simulink model "test_loopback_buf"  (Simulink 6.2)
settings: Solver=ode45  StartTime=0.0  StopTime=4000  RelTol=1e-3
undefined symbols (not defined in the file): Down, Up
libraries: xbsIndex_r3 x1383, xps_library x52, casper_library x37
(part 2 of 8)

== system test_loopback_buf/Feng_sim_complete1 ==
  Concat : xbsIndex_r3/Concat  num_inputs=2  explicit_period=off  period=1  dbl_ovrd=off
  Concat1 : xbsIndex_r3/Concat  num_inputs=3  explicit_period=off  period=1  dbl_ovrd=off
  Constant : xbsIndex_r3/Constant  const=0  equ=P=C  arith_type=Boolean  n_bits=1  bin_pt=0  opselect=C  inp2=PCIN>>17  opr=+  inp1=P  carry=CIN  iostate=0  explicit_period=on  period=1  dbl_ovrd=off
  Constant1 : xbsIndex_r3/Constant  const=1  equ=P=C  arith_type=Boolean  n_bits=1  bin_pt=0  opselect=C  inp2=PCIN>>17  opr=+  inp1=P  carry=CIN  iostate=0  explicit_period=off  period=1  dbl_ovrd=off
  Constant2 : Constant
  Constant3 : xbsIndex_r3/Constant  const=0  equ=P=C  arith_type=Boolean  n_bits=1  bin_pt=0  opselect=C  inp2=PCIN>>17  opr=+  inp1=P  carry=CIN  iostate=0  explicit_period=off  period=1  dbl_ovrd=off
  Constant4 : xbsIndex_r3/Constant  const=0  equ=P=C  arith_type=Unsigned  n_bits=32  bin_pt=0  opselect=C  inp2=PCIN>>17  opr=+  inp1=P  carry=CIN  iostate=0  explicit_period=on  period=1  dbl_ovrd=off
  Constant5 : xbsIndex_r3/Constant  const=0  equ=P=C  arith_type=Unsigned  n_bits=16-2  bin_pt=0  opselect=C  inp2=PCIN>>17  opr=+  inp1=P  carry=CIN  iostate=0  explicit_period=on  period=1  dbl_ovrd=off
  Convert1 : xbsIndex_r3/Convert  arith_type=Boolean  n_bits=8  bin_pt=6  quantization=Truncate  overflow=Wrap  latency=0  explicit_period=on  period=1  dbl_ovrd=off  show_param=off  inserted_by_tool=off  pipeline=off
      settings: xl_area=[0, 0, 0, 0, 0, 0, 0]
  Convert2 : xbsIndex_r3/Convert  arith_type=Boolean  n_bits=8  bin_pt=6  quantization=Truncate  overflow=Wrap  latency=0  explicit_period=on  period=1  dbl_ovrd=off  show_param=off  inserted_by_tool=off  pipeline=off
      settings: xl_area=[0, 0, 0, 0, 0, 0, 0]
  Convert3 : xbsIndex_r3/Convert  arith_type=Boolean  n_bits=8  bin_pt=6  quantization=Truncate  overflow=Wrap  latency=0  explicit_period=on  period=1  dbl_ovrd=off  show_param=off  inserted_by_tool=off  pipeline=off
      settings: xl_area=[0, 0, 0, 0, 0, 0, 0]
  Counter1 : xbsIndex_r3/Counter  cnt_type=Free Running  n_bits=64  bin_pt=0  arith_type=Unsigned  start_count=0  cnt_to=Inf  cnt_by_val=1  operation=Up  explicit_period=off  period=1  load_pin=off  rst=on  en=on  dbl_ovrd=off  show_param=off  use_rpm=off  gen_core=off
      settings: xl_area=[0, 0, 0, 0, 0, 0, 0]
  Counter2 : xbsIndex_r3/Counter  cnt_type=Free Running  n_bits=32  bin_pt=0  arith_type=Unsigned  start_count=1  cnt_to=Inf  cnt_by_val=1  operation=Up  explicit_period=on  period=1  load_pin=off  rst=on  en=off  dbl_ovrd=off  show_param=off  use_rpm=on  gen_core=off
      settings: xl_area=[0, 0, 0, 0, 0, 0, 0]
  Counter3 : xbsIndex_r3/Counter  cnt_type=Free Running  n_bits=32  bin_pt=0  arith_type=Unsigned  start_count=0  cnt_to=1023  cnt_by_val=1  operation=Up  explicit_period=on  period=1  load_pin=off  rst=on  en=on  dbl_ovrd=off  show_param=off  use_rpm=on  gen_core=off
      settings: xl_area=[0, 0, 0, 0, 0, 0, 0]
  Counter4 : xbsIndex_r3/Counter  cnt_type=Free Running  n_bits=2  bin_pt=0  arith_type=Unsigned  start_count=0  cnt_to=1023  cnt_by_val=1  operation=Up  explicit_period=on  period=1  load_pin=off  rst=off  en=on  dbl_ovrd=off  show_param=off  use_rpm=on  gen_core=off
      settings: xl_area=[0, 0, 0, 0, 0, 0, 0]
  Delay{1..2,4..5,8} (5 alike) : xbsIndex_r3/Delay  latency=1  reg_retiming=on  explicit_period=off  period=1  en=off  accept_only_valid=off  init_zero=on  dbl_ovrd=off  show_param=off
      settings: xl_area=[0, 0, 0, 0, 0, 0, 0]
  Gateway Out{,1..4} (5 alike) : xbsIndex_r3/Gateway Out  output_type=Double  nbits=8  bin_pt=6  arith_type=Boolean  quantization=Truncate  overflow=Wrap  hdl_port=on  timing_constraint=None  locs_specified=off  LOCs={}  needs_fixed_name=off  show_param=off
      settings: xl_area=[0, 0, 0, 0, 0, 0, 0]
  Inverter : xbsIndex_r3/Inverter  latency=0  explicit_period=off  period=1  en=off  dbl_ovrd=off  show_param=off
      settings: xl_area=[0, 0, 0, 0, 0, 0, 0]
  Inverter1 : xbsIndex_r3/Inverter  latency=0  explicit_period=off  period=1  en=off  dbl_ovrd=off  show_param=off
      settings: xl_area=[0, 0, 0, 0, 0, 0, 0]
  Inverter2 : xbsIndex_r3/Inverter  latency=0  explicit_period=off  period=1  en=off  dbl_ovrd=off  show_param=off
      settings: xl_area=[0, 0, 0, 0, 0, 0, 0]
  Logical : xbsIndex_r3/Logical  logical_function=AND  inputs=2  precision=Full  arith_type=Unsigned  n_bits=8  bin_pt=2  align_bp=on  latency=0  explicit_period=off  period=1  en=off  dbl_ovrd=off  show_param=off
      settings: xl_area=[0, 0, 0, 0, 0, 0, 0]
  Mux{,1..3} (4 alike) : xbsIndex_r3/Mux  inputs=2  precision=Full  arith_type="Signed  (2's comp)"  n_bits=8  bin_pt=2  quantization=Truncate  overflow=Wrap  latency=1  explicit_period=off  period=1  en=off  dbl_ovrd=off  show_param=off  mux_type=off  use_rpm=off  gen_core=off
      settings: xl_area=[0, 0, 0, 0, 0, 0, 0]
  Relational : xbsIndex_r3/Relational  mode=a>=b  latency=0  explicit_period=on  period=1  en=off  dbl_ovrd=off  show_param=off
      settings: xl_area=[0, 0, 0, 0, 0, 0, 0]
  Relational1 : xbsIndex_r3/Relational  mode=a=b  latency=0  explicit_period=off  period=1  en=off  dbl_ovrd=off  show_param=off
      settings: xl_area=[0, 0, 0, 0, 0, 0, 0]
  Relational5 : xbsIndex_r3/Relational  mode=a<=b  latency=0  explicit_period=off  period=1  en=off  dbl_ovrd=off  show_param=off
      settings: xl_area=[0, 0, 0, 0, 0, 0, 0]
  Scope : Scope  NumInputPorts=5
      settings: TimeRange=4000  YMin=130000~0~0~0~0  YMax=200000~1~1~1~1  SaveName=ScopeData11
  Slice : xbsIndex_r3/Slice  mode=Upper Bit Location + Width  nbits=31  bit1=0  base1=MSB of Input  bit0=0  base0=LSB of Input  boolean_output=off  explicit_period=off  period=1  dbl_ovrd=off
  Slice1 : xbsIndex_r3/Slice  mode=Lower Bit Location + Width  nbits=1  bit1=1  base1=MSB of Input  bit0=0  base0=LSB of Input  boolean_output=off  explicit_period=off  period=1  dbl_ovrd=off
  Slice2 : xbsIndex_r3/Slice  mode=Lower Bit Location + Width  nbits=2  bit1=1  base1=MSB of Input  bit0=0  base0=LSB of Input  boolean_output=off  explicit_period=off  period=1  dbl_ovrd=off
  Slice3 : xbsIndex_r3/Slice  mode=Lower Bit Location + Width  nbits=48  bit1=1  base1=MSB of Input  bit0=3  base0=LSB of Input  boolean_output=off  explicit_period=off  period=1  dbl_ovrd=off
  Slice4 : xbsIndex_r3/Slice  mode=Lower Bit Location + Width  nbits=1  bit1=1  base1=MSB of Input  bit0=1  base0=LSB of Input  boolean_output=off  explicit_period=off  period=1  dbl_ovrd=off
  ip_addr : xps_library/software register  Tag=xps:sw_reg  io_dir=From Processor  arith_type=Unsigned  bitwidth=32  bin_pt=0  sample_period=1  gw_name=test_loopback_buf_Feng_sim_complete1_ip_addr_user_data_out
  mcnt_cnt : xbsIndex_r3/Counter  cnt_type=Free Running  n_bits=64  bin_pt=0  arith_type=Unsigned  start_count=0  cnt_to=Inf  cnt_by_val=1  operation=Up  explicit_period=off  period=1  load_pin=off  rst=off  en=on  dbl_ovrd=off  show_param=off  use_rpm=off  gen_core=off
      settings: xl_area=[0, 0, 0, 0, 0, 0, 0]
  negedge : casper_library/Misc/negedge  Tag=Rising Edge Detector
  payload_len : xps_library/software register  Tag=xps:sw_reg  io_dir=From Processor  arith_type=Unsigned  bitwidth=32  bin_pt=0  sample_period=1  gw_name=test_loopback_buf_Feng_sim_complete1_payload_len_user_data_out
  period : xps_library/software register  Tag=xps:sw_reg  io_dir=From Processor  arith_type=Unsigned  bitwidth=32  bin_pt=0  sample_period=1  gw_name=test_loopback_buf_Feng_sim_complete1_period_user_data_out
  posedge : casper_library/Misc/pulse_ext/posedge  Tag=Rising Edge Detector
  run : xps_library/software register  Tag=xps:sw_reg  io_dir=From Processor  arith_type=Unsigned  bitwidth=32  bin_pt=0  sample_period=1  gw_name=test_loopback_buf_Feng_sim_complete1_run_user_data_out
  sim_IP : Constant  Value=0
  sim_freq : Constant  Value=52
  sim_length : Constant  Value=50
  d_out : Outport
  valid : Outport  Port=2
  dest_ip : Outport  Port=3
  eof : Outport  Port=4
  discard : Outport  Port=5
  wires:
  Delay1/1 -> Delay8/1
  Slice2/1 -> Concat1/3
  Slice3/1 -> Concat1/1
  Logical/1 -> Gateway Out3/1, Delay2/1
  Gateway Out4/1 -> Scope/5
  Gateway Out3/1 -> Scope/4
  Gateway Out2/1 -> Scope/3
  Gateway Out1/1 -> Scope/2
  Gateway Out/1 -> Scope/1
  Delay5/1 -> Gateway Out4/1, Mux3/1
  Concat1/1 -> Gateway Out/1, Mux3/2
  Constant5/1 -> Concat1/2
  mcnt_cnt/1 -> Slice3/1
  Inverter2/1 -> Logical/1, Delay5/1
  Relational1/1 -> Inverter2/1
  Constant4/1 -> Relational1/1
  Concat/1 -> Slice2/1, Delay1/1
  Slice/1 -> Concat/1
  Counter4/1 -> Slice4/1
  ip_addr/1 -> Slice/1
  Convert2/1 -> Delay4/1
  Inverter1/1 -> Convert2/1
  Constant1/1 -> Mux2/3
  Constant3/1 -> Mux2/2
  Convert3/1 -> Inverter/1
  Delay2/1 -> Counter1/2
  Inverter/1 -> Counter1/1
  Mux2/1 -> Mux/3
  Delay4/1 -> discard/1
  Slice1/1 -> Convert3/1, Inverter1/1, Mux1/1, Mux/1
  Constant2/1 -> run/1
  run/1 -> Slice1/1
  Delay8/1 -> dest_ip/1
  Mux3/1 -> d_out/1
  Convert1/1 -> Mux1/3
  Mux1/1 -> eof/1
  Constant/1 -> Mux1/2, Mux/2
  Mux/1 -> Gateway Out2/1, valid/1
  payload_len/1 -> Relational5/2
  sim_length/1 -> payload_len/1
  posedge/1 -> Gateway Out1/1, mcnt_cnt/1, Counter4/1, Counter3/1
  Counter3/1 -> Relational1/2, Relational5/1
  Relational5/1 -> Counter3/2, negedge/1, Mux2/1, Logical/2
  sim_IP/1 -> ip_addr/1
  sim_freq/1 -> period/1
  period/1 -> Relational/2
  negedge/1 -> Convert1/1
  Counter1/1 -> Mux3/3
  Relational/1 -> Counter2/1, posedge/1
  Counter2/1 -> Relational/1
  Slice4/1 -> Concat/2

== system test_loopback_buf/depack_it ==
  note: The first 64 bit word in a packet
      | is 48 bits of mcnt + 16 bits of antenna.
      | This circuit counts through each
      | packet, registers mcnt and ant,
      | and presents them aligned with the
      | data packet.
  din : Inport  Port=1  LatchInput=off
  we : Inport  Port=2  LatchInput=off
  eof_in : Inport  Port=3  LatchInput=off
  Constant1 : xbsIndex_r3/Constant  const=0  equ=P=C  arith_type=Unsigned  n_bits=packet_bits  bin_pt=0  opselect=C  inp2=PCIN>>17  opr=+  inp1=P  carry=CIN  iostate=0  explicit_period=on  period=1  dbl_ovrd=off
  Delay4 : xbsIndex_r3/Delay  latency=1  reg_retiming=off  explicit_period=off  period=1  en=off  accept_only_valid=off  init_zero=on  dbl_ovrd=off  show_param=off
      settings: xl_area=[0, 0, 0, 0, 0, 0, 0]
  Delay5 : xbsIndex_r3/Delay  latency=1  reg_retiming=off  explicit_period=off  period=1  en=off  accept_only_valid=off  init_zero=on  dbl_ovrd=off  show_param=off
      settings: xl_area=[0, 0, 0, 0, 0, 0, 0]
  Inverter : xbsIndex_r3/Inverter  latency=0  explicit_period=off  period=1  en=off  dbl_ovrd=off  show_param=off
      settings: xl_area=[0, 0, 0, 0, 0, 0, 0]
  Logical1 : xbsIndex_r3/Logical  logical_function=AND  inputs=2  precision=Full  arith_type=Unsigned  n_bits=8  bin_pt=2  align_bp=on  latency=0  explicit_period=off  period=1  en=off  dbl_ovrd=off  show_param=off
      settings: xl_area=[0, 0, 0, 0, 0, 0, 0]
  Logical2 : xbsIndex_r3/Logical  logical_function=AND  inputs=2  precision=Full  arith_type=Unsigned  n_bits=8  bin_pt=2  align_bp=on  latency=1  explicit_period=off  period=1  en=off  dbl_ovrd=off  show_param=off
      settings: xl_area=[0, 0, 0, 0, 0, 0, 0]
  Logical3 : xbsIndex_r3/Logical  logical_function=AND  inputs=2  precision=Full  arith_type=Unsigned  n_bits=8  bin_pt=2  align_bp=on  latency=0  explicit_period=off  period=1  en=off  dbl_ovrd=off  show_param=off
      settings: xl_area=[0, 0, 0, 0, 0, 0, 0]
  Register : xbsIndex_r3/Register  init=0  reg_only_valid=off  explicit_period=off  period=1  rst=off  en=on  out_en=off  dbl_ovrd=off  show_param=off
      settings: xl_area=[0, 0, 0, 0, 0, 0, 0]
  Relational : xbsIndex_r3/Relational  mode=a=b  latency=0  explicit_period=off  period=1  en=off  dbl_ovrd=off  show_param=off
      settings: xl_area=[0, 0, 0, 0, 0, 0, 0]
  Slice1 : xbsIndex_r3/Slice  mode=Lower Bit Location + Width  nbits=48  bit1=0  base1=MSB of Input  bit0=16  base0=LSB of Input  boolean_output=off  explicit_period=off  period=1  dbl_ovrd=off
  Slice5 : xbsIndex_r3/Slice  mode=Lower Bit Location + Width  nbits=16  bit1=0  base1=MSB of Input  bit0=0  base0=LSB of Input  boolean_output=off  explicit_period=off  period=1  dbl_ovrd=off
  payload_cnt : xbsIndex_r3/Counter  cnt_type=Count Limited  n_bits=packet_bits  bin_pt=0  arith_type=Unsigned  start_count=0  cnt_to=packet_len - 1  cnt_by_val=1  operation=Up  explicit_period=off  period=1  load_pin=off  rst=on  en=on  dbl_ovrd=off  show_param=off  use_rpm=on  gen_core=off
      settings: xl_area=[0, 0, 0, 0, 0, 0, 0]
  dout : Outport
  valid : Outport  Port=2
  eof : Outport  Port=3
  mcnt : Outport  Port=4
  ant : Outport  Port=5
  wires:
  we/1 -> Logical2/1, Logical1/2, payload_cnt/2, Logical3/2
  Constant1/1 -> Relational/2
  payload_cnt/1 -> Relational/1
  Relational/1 -> Inverter/1, Logical1/1
  Logical2/1 -> valid/1
  Logical1/1 -> Register/2
  din/1 -> Delay4/1, Register/1
  Delay4/1 -> dout/1
  Delay5/1 -> eof/1
  Register/1 -> Slice5/1, Slice1/1
  Slice1/1 -> mcnt/1
  Slice5/1 -> ant/1
  Inverter/1 -> Logical2/2
  Logical3/1 -> payload_cnt/1, Delay5/1
  eof_in/1 -> Logical3/1

== system test_loopback_buf/loopback ==
  note: Only take packets transmitted
      | to my own IP address
  din : Inport  Port=1  LatchInput=off
  we : Inport  Port=2  LatchInput=off
  dest_ip : Inport  Port=3  LatchInput=off
  eof : Inport  Port=4  LatchInput=off
  discard : Inport  Port=5  LatchInput=off
  my_ip : Inport  Port=6  LatchInput=off
  ack : Inport  Port=7  LatchInput=off
  Concat : xbsIndex_r3/Concat  num_inputs=2  explicit_period=off  period=1  dbl_ovrd=off
  Constant1 : xbsIndex_r3/Constant  const=1  equ=P=C  arith_type=Boolean  n_bits=2  bin_pt=0  opselect=C  inp2=PCIN>>17  opr=+  inp1=P  carry=CIN  iostate=0  explicit_period=on  period=1  dbl_ovrd=off
  Convert : xbsIndex_r3/Convert  arith_type=Unsigned  n_bits=1  bin_pt=0  quantization=Truncate  overflow=Wrap  latency=0  explicit_period=off  period=1  dbl_ovrd=off  show_param=off  inserted_by_tool=off  pipeline=off
      settings: xl_area=[0, 0, 0, 0, 0, 0, 0]
  Inverter1 : xbsIndex_r3/Inverter  latency=0  explicit_period=off  period=1  en=off  dbl_ovrd=off  show_param=off
      settings: xl_area=[0, 0, 0, 0, 0, 0, 0]
  Logical1 : xbsIndex_r3/Logical  logical_function=OR  inputs=2  precision=Full  arith_type=Unsigned  n_bits=8  bin_pt=2  align_bp=on  latency=0  explicit_period=off  period=1  en=off  dbl_ovrd=off  show_param=off
      settings: xl_area=[0, 0, 0, 0, 0, 0, 0]
  Logical2 : xbsIndex_r3/Logical  logical_function=AND  inputs=2  precision=Full  arith_type=Unsigned  n_bits=8  bin_pt=2  align_bp=on  latency=0  explicit_period=off  period=1  en=off  dbl_ovrd=off  show_param=off
      settings: xl_area=[0, 0, 0, 0, 0, 0, 0]
  Logical4 : xbsIndex_r3/Logical  logical_function=AND  inputs=2  precision=Full  arith_type=Unsigned  n_bits=8  bin_pt=2  align_bp=on  latency=0  explicit_period=off  period=1  en=off  dbl_ovrd=off  show_param=off
      settings: xl_area=[0, 0, 0, 0, 0, 0, 0]
  Relational1 : xbsIndex_r3/Relational  mode=a=b  latency=1  explicit_period=off  period=1  en=off  dbl_ovrd=off  show_param=off
      settings: xl_area=[0, 0, 0, 0, 0, 0, 0]
  Slice : xbsIndex_r3/Slice  mode=Upper Bit Location + Width  nbits=1  bit1=0  base1=MSB of Input  bit0=0  base0=LSB of Input  boolean_output=on  explicit_period=off  period=1  dbl_ovrd=off
  Slice1 : xbsIndex_r3/Slice  mode=Lower Bit Location + Width  nbits=64  bit1=-1  base1=MSB of Input  bit0=0  base0=LSB of Input  boolean_output=off  explicit_period=off  period=1  dbl_ovrd=off
  fwft_fifo : Subsystem
  rollback_fifo : Subsystem  mask{depth_bits=depth_bits}
      mask prompts: depth_bits "Fifo Depth (2^?):"
      mask help: A rollback fifo behaves as a normal fifo, except that data which are written in have to be "committed" before they become available for readout. Moreover, any data which are written in and have not been committed can be "discarded", and will never be made available for readout.
  dout : Outport
  valid : Outport  Port=2
  eof_out : Outport  Port=3
  wires:
  Logical2/1 -> Logical1/1
  Inverter1/1 -> Logical2/2
  discard/1 -> Logical1/2
  Logical1/1 -> rollback_fifo/4(discard)
  Convert/1 -> Concat/1
  Slice/1 -> eof_out/1
  Slice1/1 -> dout/1
  din/1 -> Concat/2
  Concat/1 -> rollback_fifo/1(din)
  Logical4/1 -> rollback_fifo/3(commit)
  we/1 -> rollback_fifo/2(we)
  eof/1 -> Logical2/1, Logical4/1, Convert/1
  Relational1/1 -> Inverter1/1, Logical4/2
  my_ip/1 -> Relational1/2
  dest_ip/1 -> Relational1/1
  rollback_fifo/1(dout) -> fwft_fifo/1(din)
  rollback_fifo/2(valid) -> fwft_fifo/2(we)
  Constant1/1 -> rollback_fifo/5(re)
  ack/1 -> fwft_fifo/3(ack)
  fwft_fifo/1(dout) -> Slice1/1, Slice/1
  fwft_fifo/2(valid) -> valid/1

== system test_loopback_buf/loopback0 ==
  note: Only take packets transmitted
      | to my own IP address
  note: MUX TWO PACKET STREAMS
      | Incomming data is buffered and only stored if it is commited (valid EOF).
      | If a discard command is received, the data is flushed.
  note: THE ACK LINE MUST REMAIN HIGH EVEN WHEN VALID GOES LOW FOR FULL-SPEED READOUT.
      |
      | This is fine for the intended purpose:
      | We read out a full packet at a time, ensuring that ack stays high until EOF is received.
      |
      | The first packet read out will have the wrong length. (the first output word will be duplicated)
  note: PACKET LENGTH SHOULD NOT BE LESS THAN 3 WORDS
  din : Inport  Port=1  LatchInput=off
  we : Inport  Port=2  LatchInput=off
  dest_ip : Inport  Port=3  LatchInput=off
  eof : Inport  Port=4  LatchInput=off
  discard : Inport  Port=5  LatchInput=off
  my_ip : Inport  Port=6  LatchInput=off
  ack : Inport  Port=7  LatchInput=off
  Concat1 : xbsIndex_r3/Concat  num_inputs=2  explicit_period=off  period=1  dbl_ovrd=off
  Constant13 : xbsIndex_r3/Constant  const=0  equ=P=C  arith_type=Boolean  n_bits=1  bin_pt=0  opselect=C  inp2=PCIN>>17  opr=+  inp1=P  carry=CIN  iostate=0  explicit_period=on  period=1  dbl_ovrd=off
  Convert : xbsIndex_r3/Convert  arith_type=Unsigned  n_bits=1  bin_pt=0  quantization=Truncate  overflow=Wrap  latency=0  explicit_period=off  period=1  dbl_ovrd=off  show_param=off  inserted_by_tool=off  pipeline=off
      settings: xl_area=[0, 0, 0, 0, 0, 0, 0]
  Delay{1..3,40} (4 alike) : xbsIndex_r3/Delay  latency=2  reg_retiming=on  explicit_period=off  period=1  en=off  accept_only_valid=off  init_zero=on  dbl_ovrd=off  show_param=off
      settings: xl_area=[0, 0, 0, 0, 0, 0, 0]
  Gateway Out{1..2,22..25,39..41} (9 alike) : xbsIndex_r3/Gateway Out  output_type=Double  nbits=8  bin_pt=6  arith_type=Boolean  quantization=Truncate  overflow=Wrap  hdl_port=on  timing_constraint=None  locs_specified=off  LOCs={}  needs_fixed_name=off  show_param=off
      settings: xl_area=[0, 0, 0, 0, 0, 0, 0]
  Inverter1 : xbsIndex_r3/Inverter  latency=0  explicit_period=off  period=1  en=off  dbl_ovrd=off  show_param=off
      settings: xl_area=[0, 0, 0, 0, 0, 0, 0]
  Logical1 : xbsIndex_r3/Logical  logical_function=OR  inputs=2  precision=Full  arith_type=Unsigned  n_bits=8  bin_pt=2  align_bp=on  latency=0  explicit_period=off  period=1  en=off  dbl_ovrd=off  show_param=off
      settings: xl_area=[0, 0, 0, 0, 0, 0, 0]
  Logical2 : xbsIndex_r3/Logical  logical_function=AND  inputs=2  precision=Full  arith_type=Unsigned  n_bits=8  bin_pt=2  align_bp=on  latency=0  explicit_period=off  period=1  en=off  dbl_ovrd=off  show_param=off
      settings: xl_area=[0, 0, 0, 0, 0, 0, 0]
  Reinterpret : xbsIndex_r3/Reinterpret  force_arith_type=on  arith_type=Unsigned  force_bin_pt=on  bin_pt=0  force_valid=on
  Relational1 : xbsIndex_r3/Relational  mode=a=b  latency=0  explicit_period=off  period=1  en=off  dbl_ovrd=off  show_param=off
      settings: xl_area=[0, 0, 0, 0, 0, 0, 0]
  buf_data3 : xbsIndex_r3/Slice  mode=Lower Bit Location + Width  nbits=64  bit1=33  base1=LSB of Input  bit0=0  base0=LSB of Input  boolean_output=off  explicit_period=off  period=1  dbl_ovrd=off
  buf_debug : Scope  NumInputPorts=9
      settings: YMin=100~0~0~0~0~0~0~0.95~0  YMax=1000~1~1~3~1000~1~1~1.05~1
  buf_eof3 : xbsIndex_r3/Slice  mode=Upper Bit Location + Width  nbits=1  bit1=64  base1=LSB of Input  bit0=0  base0=LSB of Input  boolean_output=on  explicit_period=off  period=1  dbl_ovrd=off
  data_FWFT : Subsystem  mask{depth_bits=depth_bits}
      mask prompts: depth_bits "Fifo Depth (2^?):"
      mask help: A rollback fifo behaves as a normal fifo, except that data which are written in have to be "committed" before they become available for readout. Moreover, any data which are written in and have not been committed can be "discarded", and will never be made available for readout.
      mask init:
      | fmtstr = sprintf('Depth: %d', 2^depth_bits);
      | set_param(gcb, 'AttributesFormatString', fmtstr);
      settings: AttributesFormatString=Depth: 1024
  overflow_cnt : xps_library/software register  Tag=xps:sw_reg  io_dir=To Processor  arith_type=Unsigned  bitwidth=32  bin_pt=0  sample_period=1  gw_name=b_2x_8a_r310_a_loopback0_overflow_cnt_user_data_in
  overflows : xbsIndex_r3/Counter  cnt_type=Free Running  n_bits=32  bin_pt=0  arith_type=Unsigned  start_count=0  cnt_to=Inf  cnt_by_val=1  operation=Up  explicit_period=off  period=1  load_pin=off  rst=off  en=on  dbl_ovrd=off  show_param=off  use_rpm=on  gen_core=off
      settings: xl_area=[0, 0, 0, 0, 0, 0, 0]
  valid_eof_0 : xbsIndex_r3/Logical  logical_function=AND  inputs=3  precision=Full  arith_type=Unsigned  n_bits=8  bin_pt=2  align_bp=on  latency=0  explicit_period=on  period=1  en=off  dbl_ovrd=off  show_param=off
      settings: xl_area=[0, 0, 0, 0, 0, 0, 0]
  dout : Outport
  valid : Outport  Port=2
  ip_addr : Outport  Port=3
  eof_out : Outport  Port=4
  discard_out : Outport  Port=5
  buf_over : Outport  Port=6
  buf_empt : Outport  Port=7
  wires:
  Logical2/1 -> Logical1/1
  Inverter1/1 -> Logical2/2
  discard/1 -> Logical1/2
  Logical1/1 -> Delay3/1
  Relational1/1 -> valid_eof_0/3, Inverter1/1
  Constant13/1 -> discard_out/1
  [data_empty] -> buf_empt/1
  [data_full] -> buf_over/1, overflows/1
  Concat1/1 -> Delay40/1
  data_FWFT/4(full) -> [data_full]
  din/1 -> [d_in], Reinterpret/1
  we/1 -> valid_eof_0/1, [v_in], Delay1/1
  valid_eof_0/1 -> [in_valid_eof], Delay2/1, Convert/1
  data_FWFT/1(dout) -> buf_eof3/1, buf_data3/1
  data_FWFT/2(valid) -> [v_out], valid/1
  [my_ip] -> ip_addr/1, [ip_out]
  overflows/1 -> overflow_cnt/1
  Gateway Out24/1 -> buf_debug/1
  Gateway Out22/1 -> buf_debug/2
  Gateway Out23/1 -> buf_debug/3
  Gateway Out25/1 -> buf_debug/4
  Gateway Out39/1 -> buf_debug/5
  Gateway Out41/1 -> buf_debug/6
  Gateway Out40/1 -> buf_debug/7
  data_FWFT/5(empty) -> [data_empty]
  buf_data3/1 -> [d_out], dout/1
  buf_eof3/1 -> [eof_out], eof_out/1
  Gateway Out1/1 -> buf_debug/8
  [ip_out] -> Gateway Out1/1
  [eof_out] -> Gateway Out40/1
  [v_out] -> Gateway Out41/1
  [d_out] -> Gateway Out39/1
  [dest_ip] -> Gateway Out25/1
  [d_in] -> Gateway Out24/1
  [v_in] -> Gateway Out22/1
  [in_valid_eof] -> Gateway Out23/1
  [data_ack] -> data_FWFT/5(ack)
  Gateway Out2/1 -> buf_debug/9
  [data_ack] -> Gateway Out2/1
  my_ip/1 -> [my_ip]
  [my_ip] -> Relational1/2
  ack/1 -> [data_ack]
  eof/1 -> valid_eof_0/2, Logical2/1
  dest_ip/1 -> [dest_ip]
  [dest_ip] -> Relational1/1
  Convert/1 -> Concat1/1
  Reinterpret/1 -> Concat1/2
  Delay40/1 -> data_FWFT/1(din)
  Delay1/1 -> data_FWFT/2(we)
  Delay2/1 -> data_FWFT/3(commit)
  Delay3/1 -> data_FWFT/4(discard)

== system test_loopback_buf/loopback1 ==
  note: Only take packets transmitted
      | to my own IP address
  din : Inport  Port=1  LatchInput=off
  we : Inport  Port=2  LatchInput=off
  dest_ip : Inport  Port=3  LatchInput=off
  eof : Inport  Port=4  LatchInput=off
  discard : Inport  Port=5  LatchInput=off
  my_ip : Inport  Port=6  LatchInput=off
  ack : Inport  Port=7  LatchInput=off
  Concat : xbsIndex_r3/Concat  num_inputs=2  explicit_period=off  period=1  dbl_ovrd=off
  Constant1 : xbsIndex_r3/Constant  const=1  equ=P=C  arith_type=Boolean  n_bits=2  bin_pt=0  opselect=C  inp2=PCIN>>17  opr=+  inp1=P  carry=CIN  iostate=0  explicit_period=on  period=1  dbl_ovrd=off
  Convert : xbsIndex_r3/Convert  arith_type=Unsigned  n_bits=1  bin_pt=0  quantization=Truncate  overflow=Wrap  latency=0  explicit_period=off  period=1  dbl_ovrd=off  show_param=off  inserted_by_tool=off  pipeline=off
      settings: xl_area=[0, 0, 0, 0, 0, 0, 0]
  Inverter1 : xbsIndex_r3/Inverter  latency=0  explicit_period=off  period=1  en=off  dbl_ovrd=off  show_param=off
      settings: xl_area=[0, 0, 0, 0, 0, 0, 0]
  Logical1 : xbsIndex_r3/Logical  logical_function=OR  inputs=2  precision=Full  arith_type=Unsigned  n_bits=8  bin_pt=2  align_bp=on  latency=0  explicit_period=off  period=1  en=off  dbl_ovrd=off  show_param=off
      settings: xl_area=[0, 0, 0, 0, 0, 0, 0]
  Logical2 : xbsIndex_r3/Logical  logical_function=AND  inputs=2  precision=Full  arith_type=Unsigned  n_bits=8  bin_pt=2  align_bp=on  latency=0  explicit_period=off  period=1  en=off  dbl_ovrd=off  show_param=off
      settings: xl_area=[0, 0, 0, 0, 0, 0, 0]
  Logical4 : xbsIndex_r3/Logical  logical_function=AND  inputs=2  precision=Full  arith_type=Unsigned  n_bits=8  bin_pt=2  align_bp=on  latency=0  explicit_period=off  period=1  en=off  dbl_ovrd=off  show_param=off
      settings: xl_area=[0, 0, 0, 0, 0, 0, 0]
  Relational1 : xbsIndex_r3/Relational  mode=a!=b  latency=1  explicit_period=off  period=1  en=off  dbl_ovrd=off  show_param=off
      settings: xl_area=[0, 0, 0, 0, 0, 0, 0]
  Slice : xbsIndex_r3/Slice  mode=Upper Bit Location + Width  nbits=1  bit1=0  base1=MSB of Input  bit0=0  base0=LSB of Input  boolean_output=on  explicit_period=off  period=1  dbl_ovrd=off
  Slice1 : xbsIndex_r3/Slice  mode=Lower Bit Location + Width  nbits=64  bit1=-1  base1=MSB of Input  bit0=0  base0=LSB of Input  boolean_output=off  explicit_period=off  period=1  dbl_ovrd=off
  fwft_fifo : Subsystem
  rollback_fifo : Subsystem  mask{depth_bits=depth_bits}
      mask prompts: depth_bits "Fifo Depth (2^?):"
      mask help: A rollback fifo behaves as a normal fifo, except that data which are written in have to be "committed" before they become available for readout. Moreover, any data which are written in and have not been committed can be "discarded", and will never be made available for readout.
  dout : Outport
  valid : Outport  Port=2
  eof_out : Outport  Port=3
  wires:
  fwft_fifo/2(valid) -> valid/1
  fwft_fifo/1(dout) -> Slice/1, Slice1/1
  ack/1 -> fwft_fifo/3(ack)
  Constant1/1 -> rollback_fifo/5(re)
  rollback_fifo/2(valid) -> fwft_fifo/2(we)
  rollback_fifo/1(dout) -> fwft_fifo/1(din)
  dest_ip/1 -> Relational1/1
  my_ip/1 -> Relational1/2
  Relational1/1 -> Logical4/2, Inverter1/1
  eof/1 -> Convert/1, Logical4/1, Logical2/1
  we/1 -> rollback_fifo/2(we)
  Logical4/1 -> rollback_fifo/3(commit)
  Concat/1 -> rollback_fifo/1(din)
  din/1 -> Concat/2
  Slice1/1 -> dout/1
  Slice/1 -> eof_out/1
  Convert/1 -> Concat/1
  Logical1/1 -> rollback_fifo/4(discard)
  discard/1 -> Logical1/2
  Inverter1/1 -> Logical2/2
  Logical2/1 -> Logical1/1

== system test_loopback_buf/loopback_buf ==
  note: Only take packets transmitted
      | to my own IP address
  note: MUX TWO PACKET STREAMS
      | Incomming data is buffered and only stored if it is commited (valid EOF).
      | If a discard command is received, the data is flushed.
  note: THE ACK LINE MUST REMAIN HIGH EVEN WHEN VALID GOES LOW FOR FULL-SPEED READOUT.
      |
      | This is fine for the intended purpose:
      | We read out a full packet at a time, ensuring that ack stays high until EOF is received.
      |
      | The first packet read out will have the wrong length. (the first output word will be duplicated)
  note: PACKET LENGTH SHOULD NOT BE LESS THAN 3 WORDS
  din : Inport  Port=1  LatchInput=off
  we : Inport  Port=2  LatchInput=off
  dest_ip : Inport  Port=3  LatchInput=off
  eof : Inport  Port=4  LatchInput=off
  discard : Inport  Port=5  LatchInput=off
  my_ip : Inport  Port=6  LatchInput=off
  ack : Inport  Port=7  LatchInput=off
  Concat1 : xbsIndex_r3/Concat  num_inputs=2  explicit_period=off  period=1  dbl_ovrd=off
  Constant13 : xbsIndex_r3/Constant  const=0  equ=P=C  arith_type=Boolean  n_bits=1  bin_pt=0  opselect=C  inp2=PCIN>>17  opr=+  inp1=P  carry=CIN  iostate=0  explicit_period=on  period=1  dbl_ovrd=off
  Convert : xbsIndex_r3/Convert  arith_type=Unsigned  n_bits=1  bin_pt=0  quantization=Truncate  overflow=Wrap  latency=0  explicit_period=off  period=1  dbl_ovrd=off  show_param=off  inserted_by_tool=off  pipeline=off
      settings: xl_area=[0, 0, 0, 0, 0, 0, 0]
  Gateway Out{1..2,22..25,39..41} (9 alike) : xbsIndex_r3/Gateway Out  output_type=Double  nbits=8  bin_pt=6  arith_type=Boolean  quantization=Truncate  overflow=Wrap  hdl_port=on  timing_constraint=None  locs_specified=off  LOCs={}  needs_fixed_name=off  show_param=off
      settings: xl_area=[0, 0, 0, 0, 0, 0, 0]
  Inverter1 : xbsIndex_r3/Inverter  latency=0  explicit_period=off  period=1  en=off  dbl_ovrd=off  show_param=off
      settings: xl_area=[0, 0, 0, 0, 0, 0, 0]
  Logical1 : xbsIndex_r3/Logical  logical_function=OR  inputs=2  precision=Full  arith_type=Unsigned  n_bits=8  bin_pt=2  align_bp=on  latency=0  explicit_period=off  period=1  en=off  dbl_ovrd=off  show_param=off
      settings: xl_area=[0, 0, 0, 0, 0, 0, 0]
  Logical2 : xbsIndex_r3/Logical  logical_function=AND  inputs=2  precision=Full  arith_type=Unsigned  n_bits=8  bin_pt=2  align_bp=on  latency=0  explicit_period=off  period=1  en=off  dbl_ovrd=off  show_param=off
      settings: xl_area=[0, 0, 0, 0, 0, 0, 0]
  Reinterpret : xbsIndex_r3/Reinterpret  force_arith_type=on  arith_type=Unsigned  force_bin_pt=on  bin_pt=0  force_valid=on
  Relational1 : xbsIndex_r3/Relational  mode=a=b  latency=0  explicit_period=off  period=1  en=off  dbl_ovrd=off  show_param=off
      settings: xl_area=[0, 0, 0, 0, 0, 0, 0]
  buf_data3 : xbsIndex_r3/Slice  mode=Lower Bit Location + Width  nbits=64  bit1=33  base1=LSB of Input  bit0=0  base0=LSB of Input  boolean_output=off  explicit_period=off  period=1  dbl_ovrd=off
  buf_debug : Scope  NumInputPorts=9
      settings: YMin=100~0~0~0~0~0~0~1~0  YMax=1000~1~1~3~1000~1~1~1~1
  buf_eof3 : xbsIndex_r3/Slice  mode=Upper Bit Location + Width  nbits=1  bit1=64  base1=LSB of Input  bit0=0  base0=LSB of Input  boolean_output=on  explicit_period=off  period=1  dbl_ovrd=off
  data_FWFT : Subsystem  mask{depth_bits=depth_bits}
      mask prompts: depth_bits "Fifo Depth (2^?):"
      mask help: A rollback fifo behaves as a normal fifo, except that data which are written in have to be "committed" before they become available for readout. Moreover, any data which are written in and have not been committed can be "discarded", and will never be made available for readout.
      mask init:
      | fmtstr = sprintf('Depth: %d', 2^depth_bits);
      | set_param(gcb, 'AttributesFormatString', fmtstr);
      settings: AttributesFormatString=Depth: 1024
  overflow_cnt : xps_library/software register  Tag=xps:sw_reg  io_dir=To Processor  arith_type=Unsigned  bitwidth=32  bin_pt=0  sample_period=1  gw_name=test_loopback_buf_loopback_buf_overflow_cnt_user_data_in
  overflows : xbsIndex_r3/Counter  cnt_type=Free Running  n_bits=32  bin_pt=0  arith_type=Unsigned  start_count=0  cnt_to=Inf  cnt_by_val=1  operation=Up  explicit_period=off  period=1  load_pin=off  rst=off  en=on  dbl_ovrd=off  show_param=off  use_rpm=on  gen_core=off
      settings: xl_area=[0, 0, 0, 0, 0, 0, 0]
  valid_eof_0 : xbsIndex_r3/Logical  logical_function=AND  inputs=3  precision=Full  arith_type=Unsigned  n_bits=8  bin_pt=2  align_bp=on  latency=0  explicit_period=on  period=1  en=off  dbl_ovrd=off  show_param=off
      settings: xl_area=[0, 0, 0, 0, 0, 0, 0]
  dout : Outport
  valid : Outport  Port=2
  ip_addr : Outport  Port=3
  eof_out : Outport  Port=4
  discard_out : Outport  Port=5
  buf_over : Outport  Port=6
  buf_empt : Outport  Port=7
  ack_in : Outport  Port=8
  wires:
  Logical2/1 -> Logical1/1
  Inverter1/1 -> Logical2/2
  discard/1 -> Logical1/2
  Logical1/1 -> data_FWFT/4(discard)
  Relational1/1 -> valid_eof_0/3, Inverter1/1
  Constant13/1 -> discard_out/1
  [data_empty] -> buf_empt/1
  [data_full] -> buf_over/1, overflows/1
  Concat1/1 -> data_FWFT/1(din)
  data_FWFT/4(full) -> [data_full]
  din/1 -> [d_in], Reinterpret/1
  we/1 -> valid_eof_0/1, [v_in], data_FWFT/2(we)
  data_FWFT/3(wr_ack) -> ack_in/1
  valid_eof_0/1 -> [in_valid_eof], data_FWFT/3(commit), Convert/1
  data_FWFT/1(dout) -> buf_eof3/1, buf_data3/1
  data_FWFT/2(valid) -> [v_out], valid/1
  [my_ip] -> ip_addr/1, [ip_out]
  overflows/1 -> overflow_cnt/1
  Gateway Out24/1 -> buf_debug/1
  Gateway Out22/1 -> buf_debug/2
  Gateway Out23/1 -> buf_debug/3
  Gateway Out25/1 -> buf_debug/4
  Gateway Out39/1 -> buf_debug/5
  Gateway Out41/1 -> buf_debug/6
  Gateway Out40/1 -> buf_debug/7
  data_FWFT/5(empty) -> [data_empty]
  buf_data3/1 -> [d_out], dout/1
  buf_eof3/1 -> [eof_out], eof_out/1
  Gateway Out1/1 -> buf_debug/8
  [ip_out] -> Gateway Out1/1
  [eof_out] -> Gateway Out40/1
  [v_out] -> Gateway Out41/1
  [d_out] -> Gateway Out39/1
  [dest_ip] -> Gateway Out25/1
  [d_in] -> Gateway Out24/1
  [v_in] -> Gateway Out22/1
  [in_valid_eof] -> Gateway Out23/1
  [data_ack] -> data_FWFT/5(ack)
  Gateway Out2/1 -> buf_debug/9
  [data_ack] -> Gateway Out2/1
  my_ip/1 -> [my_ip]
  [my_ip] -> Relational1/2
  ack/1 -> [data_ack]
  eof/1 -> valid_eof_0/2, Logical2/1
  dest_ip/1 -> [dest_ip]
  [dest_ip] -> Relational1/1
  Convert/1 -> Concat1/1
  Reinterpret/1 -> Concat1/2

== system test_loopback_buf/loopback_buf1 ==
  note: Only take packets transmitted
      | to my own IP address
  note: MUX TWO PACKET STREAMS
      | Incomming data is buffered and only stored if it is commited (valid EOF).
      | If a discard command is received, the data is flushed.
  note: THE ACK LINE MUST REMAIN HIGH EVEN WHEN VALID GOES LOW FOR FULL-SPEED READOUT.
      |
      | This is fine for the intended purpose:
      | We read out a full packet at a time, ensuring that ack stays high until EOF is received.
      |
      | The first packet read out will have the wrong length. (the first output word will be duplicated)
  note: PACKET LENGTH SHOULD NOT BE LESS THAN 3 WORDS
  din : Inport  Port=1  LatchInput=off
  we : Inport  Port=2  LatchInput=off
  dest_ip : Inport  Port=3  LatchInput=off
  eof : Inport  Port=4  LatchInput=off
  discard : Inport  Port=5  LatchInput=off
  my_ip : Inport  Port=6  LatchInput=off
  ack : Inport  Port=7  LatchInput=off
  Concat1 : xbsIndex_r3/Concat  num_inputs=2  explicit_period=off  period=1  dbl_ovrd=off
  Constant13 : xbsIndex_r3/Constant  const=0  equ=P=C  arith_type=Boolean  n_bits=1  bin_pt=0  opselect=C  inp2=PCIN>>17  opr=+  inp1=P  carry=CIN  iostate=0  explicit_period=on  period=1  dbl_ovrd=off
  Convert : xbsIndex_r3/Convert  arith_type=Unsigned  n_bits=1  bin_pt=0  quantization=Truncate  overflow=Wrap  latency=0  explicit_period=off  period=1  dbl_ovrd=off  show_param=off  inserted_by_tool=off  pipeline=off
      settings: xl_area=[0, 0, 0, 0, 0, 0, 0]
  Gateway Out{1..2,22..25,39..41} (9 alike) : xbsIndex_r3/Gateway Out  output_type=Double  nbits=8  bin_pt=6  arith_type=Boolean  quantization=Truncate  overflow=Wrap  hdl_port=on  timing_constraint=None  locs_specified=off  LOCs={}  needs_fixed_name=off  show_param=off
      settings: xl_area=[0, 0, 0, 0, 0, 0, 0]
  Inverter1 : xbsIndex_r3/Inverter  latency=0  explicit_period=off  period=1  en=off  dbl_ovrd=off  show_param=off
      settings: xl_area=[0, 0, 0, 0, 0, 0, 0]
  Logical1 : xbsIndex_r3/Logical  logical_function=OR  inputs=2  precision=Full  arith_type=Unsigned  n_bits=8  bin_pt=2  align_bp=on  latency=0  explicit_period=off  period=1  en=off  dbl_ovrd=off  show_param=off
      settings: xl_area=[0, 0, 0, 0, 0, 0, 0]
  Logical2 : xbsIndex_r3/Logical  logical_function=AND  inputs=2  precision=Full  arith_type=Unsigned  n_bits=8  bin_pt=2  align_bp=on  latency=0  explicit_period=off  period=1  en=off  dbl_ovrd=off  show_param=off
      settings: xl_area=[0, 0, 0, 0, 0, 0, 0]
  Reinterpret : xbsIndex_r3/Reinterpret  force_arith_type=on  arith_type=Unsigned  force_bin_pt=on  bin_pt=0  force_valid=on
  Relational1 : xbsIndex_r3/Relational  mode=a=b  latency=0  explicit_period=off  period=1  en=off  dbl_ovrd=off  show_param=off
      settings: xl_area=[0, 0, 0, 0, 0, 0, 0]
  buf_data3 : xbsIndex_r3/Slice  mode=Lower Bit Location + Width  nbits=64  bit1=33  base1=LSB of Input  bit0=0  base0=LSB of Input  boolean_output=off  explicit_period=off  period=1  dbl_ovrd=off
  buf_debug : Scope  NumInputPorts=9
      settings: YMin=100~0~0~0~0~0~0~1~0  YMax=1000~1~1~3~1000~1~1~1~1
  buf_eof3 : xbsIndex_r3/Slice  mode=Upper Bit Location + Width  nbits=1  bit1=64  base1=LSB of Input  bit0=0  base0=LSB of Input  boolean_output=on  explicit_period=off  period=1  dbl_ovrd=off
  data_FWFT : Subsystem  mask{depth_bits=depth_bits}
      mask prompts: depth_bits "Fifo Depth (2^?):"
      mask help: A rollback fifo behaves as a normal fifo, except that data which are written in have to be "committed" before they become available for readout. Moreover, any data which are written in and have not been committed can be "discarded", and will never be made available for readout.
      mask init:
      | fmtstr = sprintf('Depth: %d', 2^depth_bits);
      | set_param(gcb, 'AttributesFormatString', fmtstr);
      settings: AttributesFormatString=Depth: 1024
  overflow_cnt : xps_library/software register  Tag=xps:sw_reg  io_dir=To Processor  arith_type=Unsigned  bitwidth=32  bin_pt=0  sample_period=1  gw_name=test_loopback_buf_loopback_buf1_overflow_cnt_user_data_in
  overflows : xbsIndex_r3/Counter  cnt_type=Free Running  n_bits=32  bin_pt=0  arith_type=Unsigned  start_count=0  cnt_to=Inf  cnt_by_val=1  operation=Up  explicit_period=off  period=1  load_pin=off  rst=off  en=on  dbl_ovrd=off  show_param=off  use_rpm=on  gen_core=off
      settings: xl_area=[0, 0, 0, 0, 0, 0, 0]
  valid_eof_0 : xbsIndex_r3/Logical  logical_function=AND  inputs=3  precision=Full  arith_type=Unsigned  n_bits=8  bin_pt=2  align_bp=on  latency=0  explicit_period=on  period=1  en=off  dbl_ovrd=off  show_param=off
      settings: xl_area=[0, 0, 0, 0, 0, 0, 0]
  dout : Outport
  valid : Outport  Port=2
  ip_addr : Outport  Port=3
  eof_out : Outport  Port=4
  discard_out : Outport  Port=5
  buf_over : Outport  Port=6
  buf_empt : Outport  Port=7
  ack_in : Outport  Port=8
  wires:
  Logical2/1 -> Logical1/1
  Inverter1/1 -> Logical2/2
  discard/1 -> Logical1/2
  Logical1/1 -> data_FWFT/4(discard)
  Relational1/1 -> valid_eof_0/3, Inverter1/1
  Constant13/1 -> discard_out/1
  [data_empty] -> buf_empt/1
  [data_full] -> buf_over/1, overflows/1
  Concat1/1 -> data_FWFT/1(din)
  data_FWFT/4(full) -> [data_full]
  din/1 -> [d_in], Reinterpret/1
  we/1 -> valid_eof_0/1, [v_in], data_FWFT/2(we)
  data_FWFT/3(wr_ack) -> ack_in/1
  valid_eof_0/1 -> [in_valid_eof], data_FWFT/3(commit), Convert/1
  data_FWFT/1(dout) -> buf_eof3/1, buf_data3/1
  data_FWFT/2(valid) -> [v_out], valid/1
  [my_ip] -> ip_addr/1, [ip_out]
  overflows/1 -> overflow_cnt/1
  Gateway Out24/1 -> buf_debug/1
  Gateway Out22/1 -> buf_debug/2
  Gateway Out23/1 -> buf_debug/3
  Gateway Out25/1 -> buf_debug/4
  Gateway Out39/1 -> buf_debug/5
  Gateway Out41/1 -> buf_debug/6
  Gateway Out40/1 -> buf_debug/7
  data_FWFT/5(empty) -> [data_empty]
  buf_data3/1 -> [d_out], dout/1
  buf_eof3/1 -> [eof_out], eof_out/1
  Gateway Out1/1 -> buf_debug/8
  [ip_out] -> Gateway Out1/1
  [eof_out] -> Gateway Out40/1
  [v_out] -> Gateway Out41/1
  [d_out] -> Gateway Out39/1
  [dest_ip] -> Gateway Out25/1
  [d_in] -> Gateway Out24/1
  [v_in] -> Gateway Out22/1
  [in_valid_eof] -> Gateway Out23/1
  [data_ack] -> data_FWFT/5(ack)
  Gateway Out2/1 -> buf_debug/9
  [data_ack] -> Gateway Out2/1
  my_ip/1 -> [my_ip]
  [my_ip] -> Relational1/2
  ack/1 -> [data_ack]
  eof/1 -> valid_eof_0/2, Logical2/1
  dest_ip/1 -> [dest_ip]
  [dest_ip] -> Relational1/1
  Convert/1 -> Concat1/1
  Reinterpret/1 -> Concat1/2
